simulink model "MIL4L3_SW6_V1_20220211"  (R2018b)
settings: Solver=FixedStepAuto  StartTime=0.0  StopTime=inf  FixedStep=0.001  RelTol=1e-3
PreLoadFcn:
  | A0_MILtest;
undefined symbols (not defined in the file or in its folder): Clb_ICADirect_LaneDisp_StateFive, Clb_ICADirect_LaneDisp_StateFour, Clb_ICADirect_LaneDisp_StateOne, Clb_ICADirect_LaneDisp_StateThree, Clb_ICADirect_LaneDisp_StateTwo, Clb_ICADirect_LaneDisp_StateZero, Clb_ICADirect_LaneDispSW, Clb_ICADirect_TrnLghtsCom_Switch, Clb_ICADirect_TrnLghtsCom_Value, Clb_ICADirect_TrnLghtsCrtl_Inhb, IMAP_Clb_ACU_Driver_Belt, IMAP_Clb_ACU_Driver_Belt_Over, IMAP_Clb_ACU_Passenger_Belt, IMAP_Clb_ACU_Passenger_Belt_Over, IMAP_Clb_ACU_RearLeft_Belt, IMAP_Clb_ACU_RearLeft_Belt_Over, IMAP_Clb_ACU_RearMiddle_Belt, IMAP_Clb_ACU_RearMiddle_Belt_Over, IMAP_Clb_ACU_RearRight_Belt, IMAP_Clb_ACU_RearRight_Belt_Over, IMAP_Clb_AEB_Switch, IMAP_Clb_AEB_Switch_Over, IMAP_Clb_ALC_TLC_Mode, IMAP_Clb_ALC_TLC_Mode_Over, IMAP_Clb_BCM_Battery_Voltage, IMAP_Clb_BCM_Battery_Voltage_Over, IMAP_Clb_BCM_BrakeLamp_State, IMAP_Clb_BCM_BrakeLamp_State_Over, IMAP_Clb_BCM_CHMSL_Status, IMAP_Clb_BCM_CHMSL_Status_Over, IMAP_Clb_BCM_Door_Lock_State, IMAP_Clb_BCM_Door_Lock_State_Over, IMAP_Clb_BCM_FrontWiper_State, IMAP_Clb_BCM_FrontWiper_State_Over, IMAP_Clb_BCM_FrontWiper_Switch, IMAP_Clb_BCM_FrontWiper_Switch_Over, IMAP_Clb_BCM_HazardLamp, IMAP_Clb_BCM_HazardLamp_Over, IMAP_Clb_BCM_HazardLamp_Switch, IMAP_Clb_BCM_HazardLamp_Switch_Over, IMAP_Clb_BCM_HighBeam_State, IMAP_Clb_BCM_HighBeam_State_Over, IMAP_Clb_BCM_Ignition_State, IMAP_Clb_BCM_Ignition_State_Over, IMAP_Clb_BCM_IHBC_Enabled, IMAP_Clb_BCM_IHBC_Enabled_Over, IMAP_Clb_BCM_Left_Light, IMAP_Clb_BCM_Left_Light_Over, IMAP_Clb_BCM_LeftTurn_Switch, IMAP_Clb_BCM_LeftTurn_Switch_Over, IMAP_Clb_BCM_LF_Door_State, IMAP_Clb_BCM_LF_Door_State_Over, IMAP_Clb_BCM_LowBeam_State, IMAP_Clb_BCM_LowBeam_State_Over, IMAP_Clb_BCM_LR_Door_State, IMAP_Clb_BCM_LR_Door_State_Over, IMAP_Clb_BCM_RF_Door_State, IMAP_Clb_BCM_RF_Door_State_Over, IMAP_Clb_BCM_Right_Light, IMAP_Clb_BCM_Right_Light_Over ... (+547)
libraries: CarMaker4SL x2153, simulink x292, dspstat3 x3, canmsglib x2, simulink_extras x1
(part 12 of 52)

== system MIL4L3_SW6_V1_20220211/CarMaker/VehicleControl/FunctionDataLog/AEB ==
  Bus Selector : BusSelector  OutputSignals=IMAPve_d_AEB_Switch,IMAPve_d_FCW_Switch,IMAPve_d_FCW_Sensitivity
  Bus Selector1 : BusSelector  OutputSignals=IMAPve_g_ESC_LatAcc,IMAPve_g_ESC_YawRate,IMAPve_d_ESC_YawRate_Valid,IMAPve_g_ESC_VehSpd,IMAPve_g_ESC_LonAcc,IMAPve_d_ESC_LonAcc_Valid,IMAPve_g_ESC_Brake_Press,IMAPve_g_ESC_Static_Slope,IMAPve_g_ESC_DySlope_Accuracy,IMAPve_g_ESC_DySlope
  Bus Selector10 : BusSelector  OutputSignals=IMAPve_d_ESC_ABS_Valid
  Bus Selector11 : BusSelector  OutputSignals=IMAPve_d_EMS_AccPedal_Fault
  Bus Selector2 : BusSelector  OutputSignals=IMAPve_g_SW_Angle,IMAPve_g_SW_Angle_Speed
  Bus Selector3 : BusSelector  OutputSignals=IMAPve_d_BCM_Left_Light,IMAPve_d_BCM_Right_Light,IMAPve_d_BCM_Opening_State
  Bus Selector4 : BusSelector  OutputSignals=IMAPve_g_EMS_RealPedal,IMAPve_d_ESC_Veh_Standstill,IMAPve_d_TCU_Actual_Gear
  Bus Selector5 : BusSelector  OutputSignals=IMAPve_d_BCM_Ignition_State,IMAPve_d_ACU_Driver_Belt,IMAPve_d_SWS_Fault_Code,IMAPve_d_SWS_Failure_Status,IMAPve_d_ESC_OFF,IMAPve_d_ESC_AlarmSig,IMAPve_d_ESC_ESC_Active,IMAPve_d_ESC_MSR_Active,IMAPve_d_ESC_TCS_Active,IMAPve_d_ESC_VehSpd_Valid,IMAPve_d_Brake_Pedal_Fault,IMAPve_d_ESC_ABS_Active,IMAPve_d_ESC_FL_WheelPulVal,IMAPve_d_ESC_FR_WheelPulVal,IMAPve_d_ESC_RL_WheelPulVal,IMAPve_d_ESC_RR_WheelPulVal,IMAPve_d_TCU_AT_Failure,IMAPve_d_EMS_Engine_Status,IMAPve_d_ESC_AEB_Status,IMAPve_d_ESC_AEB_Available,IMAPve_d_ESC_AEB_Active,IMAPve_d_BCM_FrontWiper_State,IMAPve_d_BCM_CHMSL_Status,IMAPve_d_BCM_BrakeLamp_State,IMAPve_d_ACU_Passenger_Belt,IMAPve_d_EMS_Brake_Pedal,IMAPve_d_EPB_Status,IMAPve_d_ESC_Drive_Direction,IMAPve_d_ESC_Hold_State,IMAPve_d_Radar_State,IMAPve_d_Signal_Time_Stamp,IMAPve_d_Time_System_Clock
  Bus Selector6 : BusSelector  OutputSignals=IMAPve_d_Sensor_Status,IMAPve_d_LF_Radar_Status,IMAPve_d_RF_Radar_Status,IMAPve_d_LR_Radar_Status,IMAPve_d_RR_Radar_Status,IMAPve_d_Fusion_Status,IMAPve_g_Fusion_Time_Stamp,IMAPve_d_obj_Num,IMAPva_d_obj_id,IMAPva_g_obj_pos_x,IMAPva_g_obj_pos_y,IMAPva_g_obj_vel_x,IMAPva_g_obj_vel_y,IMAPva_g_obj_acc_x,IMAPva_g_obj_acc_y,IMAPva_g_obj_pos_var_x,IMAPva_g_obj_pos_var_y,IMAPva_g_obj_pos_var_xy,IMAPva_g_obj_width,IMAPva_g_obj_length,IMAPva_d_obj_class,IMAPva_d_obj_lane,IMAPva_d_obj_status,IMAPva_d_obj_age,IMAPva_d_obj_TurnLight,IMAPva_d_obj_BrakeLight,IMAPva_d_obj_MotionStatus,IMAPve_d_Camera_Signal_Fault,IMAPve_d_Radar_Status,IMAPve_d_Camera_Status
  Bus Selector7 : BusSelector  OutputSignals=FDMMve_d_AebFcnConf,FDMMve_d_SignalTStamp
  Bus Selector8 : BusSelector  Commented=on  OutputSignals=JABSve_d_Switching,JABSve_a_DecelReq,JABSve_d_FltStatus,JABSve_d_AlertReq,JABSve_d_HapticAlarm,JABSve_d_Tips,JABSve_d_DbSignalTStamp
  Bus Selector9 : BusSelector  OutputSignals=IMAPve_d_ORI_CIPV_ID,IMAPve_d_ORI_Obj_Num,IMAPva_g_ORI_Probability,IMAPva_d_ORI_Obj_Class,IMAPva_d_ORI_Obj_Motion,IMAPva_g_ORI_Obj_RelVel,IMAPva_g_ORI_Obj_LongDis,IMAPva_d_ORI_Obj_Lane,IMAPva_g_ORI_Obj_LAngle,IMAPva_g_ORI_Obj_RAngle,IMAPva_g_ORI_Obj_Width,IMAPva_d_ORI_Obj_ID
  BusCreator : BusCreator  Inputs=109
  Data Type Conversion{,1..23,27..32} (30 alike) : DataTypeConversion
  From21 : From  Commented=on  GotoTag=JA_output
  Ground : Ground
  To Workspace : ToWorkspace  VariableName=AEBDataLog  SaveFormat=Timeseries  SampleTime=-1
  wires:
  [MDD_deceleration_type] -> BusCreator/107
  Bus Selector11/1 -> BusCreator/109  "<IMAPve_d_EMS_AccPedal_Fault>"
  [IMAP_bsPTState] -> Bus Selector11/1
  [IMAP_State] -> Bus Selector10/1
  Bus Selector9/12 -> BusCreator/105  "<IMAPva_d_ORI_Obj_ID>"
  Bus Selector9/11 -> BusCreator/104  "<IMAPva_g_ORI_Obj_Width>"
  Bus Selector9/10 -> BusCreator/103  "<IMAPva_g_ORI_Obj_RAngle>"
  Bus Selector9/9 -> BusCreator/102  "<IMAPva_g_ORI_Obj_LAngle>"
  Bus Selector9/8 -> BusCreator/101  "<IMAPva_d_ORI_Obj_Lane>"
  Bus Selector9/7 -> BusCreator/100  "<IMAPva_g_ORI_Obj_LongDis>"
  Bus Selector9/6 -> BusCreator/99  "<IMAPva_g_ORI_Obj_RelVel>"
  Bus Selector9/5 -> BusCreator/98  "<IMAPva_d_ORI_Obj_Motion>"
  Bus Selector9/4 -> BusCreator/97  "<IMAPva_d_ORI_Obj_Class>"
  Bus Selector9/3 -> BusCreator/96  "<IMAPva_g_ORI_Probability>"
  Bus Selector9/2 -> BusCreator/95  "<IMAPve_d_ORI_Obj_Num>"
  Bus Selector9/1 -> BusCreator/94  "<IMAPve_d_ORI_CIPV_ID>"
  [IMAP_ORI_obj] -> Bus Selector9/1
  [IMAPve_d_APA_AutoPark_WorkSt] -> BusCreator/108  "IMAPve_d_APA_AutoPark_WorkSt"
  Bus Selector10/1 -> BusCreator/106  "<IMAPve_d_ESC_ABS_Valid>"
  Bus Selector8/7 -> BusCreator/90  "<JABSve_d_DbSignalTStamp>"
  Ground/1 -> BusCreator/93
  Bus Selector7/2 -> BusCreator/92  "<FDMMve_d_SignalTStamp>"
  Bus Selector7/1 -> BusCreator/91  "<FDMMve_d_AebFcnConf>"
  Bus Selector8/6 -> BusCreator/89  "<JABSve_d_Tips>"
  Bus Selector8/5 -> BusCreator/88  "<JABSve_d_HapticAlarm>"
  Bus Selector8/4 -> BusCreator/87  "<JABSve_d_AlertReq>"
  Bus Selector8/3 -> BusCreator/86  "<JABSve_d_FltStatus>"
  Data Type Conversion32/1 -> BusCreator/83
  Bus Selector6/30 -> Data Type Conversion32/1  "<IMAPve_d_Camera_Status>"
  Data Type Conversion31/1 -> BusCreator/82
  Bus Selector6/29 -> Data Type Conversion31/1  "<IMAPve_d_Radar_Status>"
  Data Type Conversion30/1 -> BusCreator/81
  Bus Selector6/28 -> Data Type Conversion30/1  "<IMAPve_d_Camera_Signal_Fault>"
  Data Type Conversion29/1 -> BusCreator/80
  Bus Selector6/27 -> Data Type Conversion29/1  "<IMAPva_d_obj_MotionStatus>"
  Data Type Conversion28/1 -> BusCreator/79
  Bus Selector6/26 -> Data Type Conversion28/1  "<IMAPva_d_obj_BrakeLight>"
  Data Type Conversion27/1 -> BusCreator/78
  Bus Selector6/25 -> Data Type Conversion27/1  "<IMAPva_d_obj_TurnLight>"
  Data Type Conversion23/1 -> BusCreator/77
  Data Type Conversion22/1 -> BusCreator/76
  Data Type Conversion21/1 -> BusCreator/75
  Data Type Conversion20/1 -> BusCreator/74
  Data Type Conversion19/1 -> BusCreator/73
  Data Type Conversion18/1 -> BusCreator/72
  Data Type Conversion17/1 -> BusCreator/71
  Data Type Conversion16/1 -> BusCreator/70
  Data Type Conversion15/1 -> BusCreator/69
  Data Type Conversion14/1 -> BusCreator/68
  Data Type Conversion13/1 -> BusCreator/67
  Data Type Conversion12/1 -> BusCreator/66
  Data Type Conversion11/1 -> BusCreator/65
  Data Type Conversion10/1 -> BusCreator/64
  Data Type Conversion9/1 -> BusCreator/63
  Data Type Conversion8/1 -> BusCreator/62
  Data Type Conversion7/1 -> BusCreator/61
  Data Type Conversion6/1 -> BusCreator/60
  Data Type Conversion5/1 -> BusCreator/59
  Data Type Conversion4/1 -> BusCreator/58
  Data Type Conversion3/1 -> BusCreator/57
  Data Type Conversion2/1 -> BusCreator/56
  Data Type Conversion1/1 -> BusCreator/55
  Data Type Conversion/1 -> BusCreator/54
  Bus Selector5/32 -> BusCreator/53  "<IMAPve_d_Time_System_Clock>"
  Bus Selector5/31 -> BusCreator/52  "<IMAPve_d_Signal_Time_Stamp>"
  Bus Selector5/30 -> BusCreator/51  "<IMAPve_d_Radar_State>"
  Bus Selector5/29 -> BusCreator/50  "<IMAPve_d_ESC_Hold_State>"
  Bus Selector5/28 -> BusCreator/49  "<IMAPve_d_ESC_Drive_Direction>"
  Bus Selector5/27 -> BusCreator/48  "<IMAPve_d_EPB_Status>"
  Bus Selector5/26 -> BusCreator/47  "<IMAPve_d_EMS_Brake_Pedal>"
  Bus Selector5/25 -> BusCreator/46  "<IMAPve_d_ACU_Passenger_Belt>"
  Bus Selector5/24 -> BusCreator/45  "<IMAPve_d_BCM_BrakeLamp_State>"
  Bus Selector5/23 -> BusCreator/44  "<IMAPve_d_BCM_CHMSL_Status>"
  Bus Selector5/22 -> BusCreator/43  "<IMAPve_d_BCM_FrontWiper_State>"
  Bus Selector5/21 -> BusCreator/42  "<IMAPve_d_ESC_AEB_Active>"
  Bus Selector5/20 -> BusCreator/41  "<IMAPve_d_ESC_AEB_Available>"
  Bus Selector5/19 -> BusCreator/40  "<IMAPve_d_ESC_AEB_Status>"
  Bus Selector5/18 -> BusCreator/39  "<IMAPve_d_EMS_Engine_Status>"
  Bus Selector5/17 -> BusCreator/38  "<IMAPve_d_TCU_AT_Failure>"
  Bus Selector5/16 -> BusCreator/37  "<IMAPve_d_ESC_RR_WheelPulVal>"
  Bus Selector5/15 -> BusCreator/36  "<IMAPve_d_ESC_RL_WheelPulVal>"
  Bus Selector5/14 -> BusCreator/35  "<IMAPve_d_ESC_FR_WheelPulVal>"
  Bus Selector5/13 -> BusCreator/34  "<IMAPve_d_ESC_FL_WheelPulVal>"
  Bus Selector5/12 -> BusCreator/33  "<IMAPve_d_ESC_ABS_Active>"
  Bus Selector5/10 -> BusCreator/31  "<IMAPve_d_ESC_VehSpd_Valid>"
  Bus Selector5/11 -> BusCreator/32  "<IMAPve_d_Brake_Pedal_Fault>"
  Bus Selector5/9 -> BusCreator/30  "<IMAPve_d_ESC_TCS_Active>"
  Bus Selector5/8 -> BusCreator/29  "<IMAPve_d_ESC_MSR_Active>"
  Bus Selector5/7 -> BusCreator/28  "<IMAPve_d_ESC_ESC_Active>"
  Bus Selector5/6 -> BusCreator/27  "<IMAPve_d_ESC_AlarmSig>"
  Bus Selector5/5 -> BusCreator/26  "<IMAPve_d_ESC_OFF>"
  Bus Selector5/4 -> BusCreator/25  "<IMAPve_d_SWS_Failure_Status>"
  Bus Selector5/3 -> BusCreator/24  "<IMAPve_d_SWS_Fault_Code>"
  Bus Selector5/2 -> BusCreator/23  "<IMAPve_d_ACU_Driver_Belt>"
  Bus Selector5/1 -> BusCreator/22  "<IMAPve_d_BCM_Ignition_State>"
  Bus Selector4/3 -> BusCreator/21  "<IMAPve_d_TCU_Actual_Gear>"
  Bus Selector4/2 -> BusCreator/20  "<IMAPve_d_ESC_Veh_Standstill>"
  Bus Selector4/1 -> BusCreator/19  "<IMAPve_g_EMS_RealPedal>"
  Bus Selector3/3 -> BusCreator/18  "<IMAPve_d_BCM_Opening_State>"
  Bus Selector3/2 -> BusCreator/17  "<IMAPve_d_BCM_Right_Light>"
  Bus Selector3/1 -> BusCreator/16  "<IMAPve_d_BCM_Left_Light>"
  Bus Selector2/2 -> BusCreator/15  "<IMAPve_g_SW_Angle_Speed>"
  Bus Selector2/1 -> BusCreator/14  "<IMAPve_g_SW_Angle>"
  Bus Selector1/10 -> BusCreator/13  "<IMAPve_g_ESC_DySlope>"
  Bus Selector1/9 -> BusCreator/12  "<IMAPve_g_ESC_DySlope_Accuracy>"
  Bus Selector1/8 -> BusCreator/11  "<IMAPve_g_ESC_Static_Slope>"
  Bus Selector1/7 -> BusCreator/10  "<IMAPve_g_ESC_Brake_Press>"
  Bus Selector1/6 -> BusCreator/9  "<IMAPve_d_ESC_LonAcc_Valid>"
  Bus Selector1/5 -> BusCreator/8  "<IMAPve_g_ESC_LonAcc>"
  Bus Selector1/4 -> BusCreator/7  "<IMAPve_g_ESC_VehSpd>"
  Bus Selector6/13 -> Data Type Conversion12/1  "<IMAPva_g_obj_vel_y>"
  Bus Selector6/12 -> Data Type Conversion11/1  "<IMAPva_g_obj_vel_x>"
  Bus Selector6/11 -> Data Type Conversion10/1  "<IMAPva_g_obj_pos_y>"
  Bus Selector6/10 -> Data Type Conversion9/1  "<IMAPva_g_obj_pos_x>"
  Bus Selector6/9 -> Data Type Conversion8/1  "<IMAPva_d_obj_id>"
  Bus Selector6/8 -> Data Type Conversion7/1  "<IMAPve_d_obj_Num>"
  Bus Selector6/7 -> Data Type Conversion6/1  "<IMAPve_g_Fusion_Time_Stamp>"
  Bus Selector6/6 -> Data Type Conversion5/1  "<IMAPve_d_Fusion_Status>"
  Bus Selector6/5 -> Data Type Conversion4/1  "<IMAPve_d_RR_Radar_Status>"
  Bus Selector6/4 -> Data Type Conversion3/1  "<IMAPve_d_LR_Radar_Status>"
  Bus Selector6/14 -> Data Type Conversion13/1  "<IMAPva_g_obj_acc_x>"
  Bus Selector6/15 -> Data Type Conversion14/1  "<IMAPva_g_obj_acc_y>"
  Bus Selector6/16 -> Data Type Conversion15/1  "<IMAPva_g_obj_pos_var_x>"
  Bus Selector6/17 -> Data Type Conversion16/1  "<IMAPva_g_obj_pos_var_y>"
  Bus Selector6/18 -> Data Type Conversion17/1  "<IMAPva_g_obj_pos_var_xy>"
  Bus Selector6/19 -> Data Type Conversion18/1  "<IMAPva_g_obj_width>"
  Bus Selector6/20 -> Data Type Conversion19/1  "<IMAPva_g_obj_length>"
  Bus Selector6/21 -> Data Type Conversion20/1  "<IMAPva_d_obj_class>"
  Bus Selector6/22 -> Data Type Conversion21/1  "<IMAPva_d_obj_lane>"
  Bus Selector6/23 -> Data Type Conversion22/1  "<IMAPva_d_obj_status>"
  Bus Selector6/24 -> Data Type Conversion23/1  "<IMAPva_d_obj_age>"
  Bus Selector6/3 -> Data Type Conversion2/1  "<IMAPve_d_RF_Radar_Status>"
  Bus Selector6/2 -> Data Type Conversion1/1  "<IMAPve_d_LF_Radar_Status>"
  Bus Selector6/1 -> Data Type Conversion/1  "<IMAPve_d_Sensor_Status>"
  Bus Selector1/3 -> BusCreator/6  "<IMAPve_d_ESC_YawRate_Valid>"
  Bus Selector1/2 -> BusCreator/5  "<IMAPve_g_ESC_YawRate>"
  Bus Selector1/1 -> BusCreator/4  "<IMAPve_g_ESC_LatAcc>"
  From21/1 -> Bus Selector8/1
  [FDMM_output] -> Bus Selector7/1
  [IMAP_Fusion_Sig] -> Bus Selector6/1
  [IMAP_State] -> Bus Selector5/1
  [IMAP_bsPTState] -> Bus Selector4/1
  [IMAP_BESRx] -> Bus Selector3/1
  [IMAP_SWARx] -> Bus Selector2/1
  [IMAP_VehMovRx] -> Bus Selector1/1
  [IMAP_MP5Rx] -> Bus Selector/1
  Bus Selector/3 -> BusCreator/3  "<IMAPve_d_FCW_Sensitivity>"
  Bus Selector/2 -> BusCreator/2  "<IMAPve_d_FCW_Switch>"
  Bus Selector8/2 -> BusCreator/85  "<JABSve_a_DecelReq>"
  Bus Selector8/1 -> BusCreator/84  "<JABSve_d_Switching>"
  Bus Selector/1 -> BusCreator/1  "<IMAPve_d_AEB_Switch>"
  BusCreator/1 -> To Workspace/1

== system MIL4L3_SW6_V1_20220211/CarMaker/VehicleControl/FunctionDataLog/ELK ==
  Bus Selector : BusSelector  OutputSignals=IMAPve_d_LKA_Mode,IMAPve_d_ELK_Switch
  Bus Selector1 : BusSelector  OutputSignals=IMAPve_g_EMS_RealPedal,IMAPve_d_TCU_Actual_Gear,IMAPve_d_TCU_Target_Gear
  Bus Selector10 : BusSelector  OutputSignals=IMAPve_g_SW_Angle,IMAPve_g_SW_Angle_Speed
  Bus Selector11 : BusSelector  OutputSignals=IMAPve_g_ESC_LatAcc,IMAPve_g_ESC_YawRate,IMAPve_g_ESC_UnYawRate,IMAPve_g_ESC_VehSpd,IMAPve_g_ESC_LonAcc,IMAPve_g_ESC_Brake_Press
  Bus Selector12 : BusSelector  OutputSignals=IMAPve_d_BCM_Ignition_State,IMAPve_d_ACU_Driver_Belt,IMAPve_d_SWS_Fault_Code,IMAPve_d_SWS_Failure_Status,IMAPve_d_ESC_OFF,IMAPve_d_ESC_AlarmSig,IMAPve_d_ESC_ESC_Active,IMAPve_d_ESC_MSR_Active,IMAPve_d_ESC_TCS_Active,IMAPve_d_ESC_ABS_Active,IMAPve_d_ESC_FL_WheelPulVal,IMAPve_d_ESC_FR_WheelPulVal,IMAPve_d_ESC_RL_WheelPulVal,IMAPve_d_ESC_RR_WheelPulVal,IMAPve_d_ESC_AEB_Active,IMAPve_d_BCM_FrontWiper_State,IMAPve_d_BCM_HighBeam_State,IMAPve_d_ESC_Drive_Direction,IMAPve_d_EPS_Steer_Hold_State,IMAPve_d_Time_System_Clock
  Bus Selector13 : BusSelector  OutputSignals=IMAPva_g_ORI_Obj_AbsAx,IMAPva_g_ORI_Obj_AbsAy,IMAPva_g_ORI_Obj_RelVely,IMAPva_g_ORI_Obj_LateralDis,IMAPva_g_ORI_Obj_ExistProb,IMAPva_g_ORI_Obj_ClassProb,IMAPve_d_ORI_L0_ID,IMAPve_g_ORI_L0_ExistProb,IMAPve_g_ORI_L0_TypeConf,IMAPve_d_ORI_R0_ID,IMAPve_g_ORI_R0_ExistProb,IMAPve_g_ORI_R0_TypeConf,IMAPve_d_ORI_L1_ID,IMAPve_g_ORI_L1_ExistProb,IMAPve_g_ORI_L1_TypeConf,IMAPve_d_ORI_R1_ID,IMAPve_g_ORI_R1_ExistProb,IMAPve_g_ORI_R1_TypeConf,IMAPve_d_ORI_RoadedgeL0_ID,IMAPve_g_ORI_RoadedgeL0_ExistProb,IMAPve_g_ORI_RoadedgeL0_C1,IMAPve_g_ORI_RoadedgeL0_C0,IMAPve_g_ORI_RoadedgeL0_C3,IMAPve_g_ORI_RoadedgeL0_C2,IMAPve_d_ORI_RoadedgeL0_Type,IMAPve_g_ORI_RoadedgeR0_C1,IMAPve_g_ORI_RoadedgeR0_C0,IMAPve_g_ORI_RoadedgeR0_C3,IMAPve_g_ORI_RoadedgeR0_C2,IMAPve_d_ORI_RoadedgeR0_Type
  Bus Selector2 : BusSelector  OutputSignals=IMAPve_d_ORI_CIPV_ID,IMAPve_d_ORI_Obj_Num,IMAPva_g_ORI_Probability,IMAPva_d_ORI_Obj_Class,IMAPva_d_ORI_Obj_Motion,IMAPva_g_ORI_Obj_RelVel,IMAPva_g_ORI_Obj_LongDis,IMAPva_d_ORI_Obj_Lane,IMAPva_g_ORI_Obj_LAngle,IMAPva_g_ORI_Obj_RAngle,IMAPva_g_ORI_Obj_Width,IMAPva_d_ORI_Obj_ID
  Bus Selector3 : BusSelector  OutputSignals=IMAPve_d_ORI_Lane_Valid,IMAPve_d_ORI_Lane_ConsArea,IMAPve_d_ORI_Lane_RoadType,IMAPve_g_ORI_L0_C3,IMAPve_g_ORI_L0_C2,IMAPve_g_ORI_L0_C1,IMAPve_g_ORI_L0_C0,IMAPve_d_ORI_L0_Q,IMAPve_d_ORI_L0_Type,IMAPve_g_ORI_L0_VR,IMAPve_g_ORI_L0_TLC,IMAPve_g_ORI_L0_W,IMAPve_d_ORI_L0_LC,IMAPve_g_ORI_L1_C3,IMAPve_g_ORI_L1_C2,IMAPve_g_ORI_L1_C1,IMAPve_g_ORI_L1_C0,IMAPve_d_ORI_L1_Q,IMAPve_d_ORI_L1_Type,IMAPve_g_ORI_L1_VR,IMAPve_g_ORI_L1_TLC,IMAPve_g_ORI_L1_W,IMAPve_d_ORI_L1_LC,IMAPve_g_ORI_R0_C3,IMAPve_g_ORI_R0_C2,IMAPve_g_ORI_R0_C1,IMAPve_g_ORI_R0_C0,IMAPve_d_ORI_R0_Q,IMAPve_d_ORI_R0_LT,IMAPve_g_ORI_R0_VR,IMAPve_g_ORI_R0_TLC,IMAPve_g_ORI_R0_W,IMAPve_d_ORI_R0_LC,IMAPve_g_ORI_R1_C3,IMAPve_g_ORI_R1_C2,IMAPve_g_ORI_R1_C1,IMAPve_g_ORI_R1_C0,IMAPve_d_ORI_R1_Q,IMAPve_d_ORI_R1_LT,IMAPve_g_ORI_R1_VR,IMAPve_g_ORI_R1_TLC,IMAPve_g_ORI_R1_W,IMAPve_d_ORI_R1_LC
  Bus Selector4 : BusSelector  OutputSignals=IMAPve_d_Sensor_Status,IMAPve_d_LF_Radar_Status,IMAPve_d_RF_Radar_Status,IMAPve_d_LR_Radar_Status,IMAPve_d_RR_Radar_Status,IMAPve_d_Fusion_Status,IMAPve_g_Fusion_Time_Stamp,IMAPve_d_obj_Num,IMAPva_d_obj_id,IMAPva_g_obj_pos_x,IMAPva_g_obj_pos_y,IMAPva_g_obj_vel_x,IMAPva_g_obj_vel_y,IMAPva_g_obj_acc_x,IMAPva_g_obj_acc_y,IMAPva_g_obj_pos_var_x,IMAPva_g_obj_pos_var_y,IMAPva_g_obj_pos_var_xy,IMAPva_g_obj_width,IMAPva_g_obj_length,IMAPva_d_obj_class,IMAPva_d_obj_lane,IMAPva_d_obj_status,IMAPva_d_obj_TurnLight,IMAPva_d_obj_BrakeLight,IMAPva_d_obj_MotionStatus,IMAPve_d_Lane_Valid,IMAPve_d_Road_Type,IMAPve_d_ConsArea,IMAPve_g_L0_C0,IMAPve_g_L0_C1,IMAPve_g_L0_C2,IMAPve_g_L0_C3,IMAPve_g_L0_VR,IMAPve_d_L0_Q,IMAPve_d_L0_Type,IMAPve_g_L0_Confidence,IMAPve_g_L0_W,IMAPve_g_L0_TLC,IMAPve_d_L0_LC,IMAPve_g_R0_C0,IMAPve_g_R0_C1,IMAPve_g_R0_C2,IMAPve_g_R0_C3,IMAPve_g_R0_VR,IMAPve_d_R0_Q,IMAPve_d_R0_Type,IMAPve_g_R0_Confidence,IMAPve_g_R0_W,IMAPve_g_R0_TLC,IMAPve_d_R0_LC,IMAPve_g_L1_C0,IMAPve_g_L1_C1,IMAPve_g_L1_C2,IMAPve_g_L1_C3,IMAPve_g_L1_VR,IMAPve_d_L1_Q,IMAPve_d_L1_Type,IMAPve_g_L1_Confidence,IMAPve_g_L1_W,IMAPve_g_L1_TLC,IMAPve_d_L1_LC,IMAPve_g_R1_C0,IMAPve_g_R1_C1,IMAPve_g_R1_C2,IMAPve_g_R1_C3,IMAPve_g_R1_VR,IMAPve_d_R1_Q,IMAPve_d_R1_Type,IMAPve_g_R1_Confidence,IMAPve_g_R1_W,IMAPve_g_R1_TLC,IMAPve_d_R1_LC,IMAPve_g_L0_C0_Back,IMAPve_g_L0_C1_Back,IMAPve_g_L0_C2_Back,IMAPve_g_L0_C3_Back,IMAPve_g_L0_Range_Back,IMAPve_g_L0_C0_FR_Pred,IMAPve_g_L0_C1_FR_Pred,IMAPve_g_L0_C2_FR_Pred,IMAPve_g_L0_Range_FR_Pred,IMAPve_g_R0_C0_Back,IMAPve_g_R0_C1_Back,IMAPve_g_R0_C2_Back,IMAPve_g_R0_C3_Back,IMAPve_g_R0_Range_Back,IMAPve_g_R0_C0_FR_Pred,IMAPve_g_R0_C1_FR_Pred,IMAPve_g_R0_C2_FR_Pred,IMAPve_g_R0_Range_FR_Pred,IMAPve_g_L1_C0_Back,IMAPve_g_L1_C1_Back,IMAPve_g_L1_C2_Back,IMAPve_g_L1_C3_Back,IMAPve_g_L1_Range_Back,IMAPve_g_L1_C0_FR_Pred,IMAPve_g_L1_C1_FR_Pred,IMAPve_g_L1_C2_FR_Pred,IMAPve_g_L1_Range_FR_Pred,IMAPve_g_R1_C0_Back,IMAPve_g_R1_C1_Back,IMAPve_g_R1_C2_Back,IMAPve_g_R1_C3_Back,IMAPve_g_R1_Range_Back,IMAPve_g_R1_C0_FR_Pred,IMAPve_g_R1_C1_FR_Pred,IMAPve_g_R1_C2_FR_Pred,IMAPve_g_R1_Range_FR_Pred,IMAPve_d_Sign_ISA_Value,IMAPve_d_TSR_Sign_Type,IMAPve_d_Camera_Signal_Fault,IMAPve_d_Radar_Status,IMAPve_d_Camera_Status
  Bus Selector5 : BusSelector  OutputSignals=IMAPve_d_EPS_SteeringAngle_Flag,IMAPve_g_EPS_SteeringAngle,IMAPve_d_EPS_Driver_Override,IMAPve_d_EPS_Driver_Active_ESA
  Bus Selector6 : BusSelector  OutputSignals=FDMMve_d_ElkFcnConf,FDMMve_d_SignalTStamp
  Bus Selector7 : BusSelector  OutputSignals=IMAPve_d_Signal_Time_Stamp
  Bus Selector8 : BusSelector  OutputSignals=IMAPve_d_EPS_LKA_State,IMAPve_g_EPS_SW_Trq,IMAPve_d_EPS_Error_State
  Bus Selector9 : BusSelector  OutputSignals=IMAPve_d_BCM_HazardLamp,IMAPve_d_BCM_Left_Light,IMAPve_d_BCM_Right_Light,IMAPve_d_BCM_Opening_State
  BusCreator : BusCreator  Inputs=249
  Constant : Constant  Commented=on  Value=0
  Constant1 : Constant  Commented=on  Value=0
  Constant2 : Constant  Commented=on  Value=0
  Data Type Conversion : DataTypeConversion  Commented=on
  Data Type Conversion1 : DataTypeConversion  Commented=on
  Data Type Conversion2 : DataTypeConversion  Commented=on
  Ground : Ground
  Ground1 : Ground
  To Workspace : ToWorkspace  VariableName=ELKDataLog  SaveFormat=Timeseries  SampleTime=-1
  wires:
  Ground1/1 -> BusCreator/249  "Runable_functionstep"
  Bus Selector13/30 -> BusCreator/248  "<IMAPve_d_ORI_RoadedgeR0_Type>"
  Bus Selector13/29 -> BusCreator/247  "<IMAPve_g_ORI_RoadedgeR0_C2>"
  Bus Selector13/28 -> BusCreator/246  "<IMAPve_g_ORI_RoadedgeR0_C3>"
  Bus Selector13/27 -> BusCreator/245  "<IMAPve_g_ORI_RoadedgeR0_C0>"
  Bus Selector13/26 -> BusCreator/244  "<IMAPve_g_ORI_RoadedgeR0_C1>"
  Bus Selector13/25 -> BusCreator/243  "<IMAPve_d_ORI_RoadedgeL0_Type>"
  Bus Selector13/24 -> BusCreator/242  "<IMAPve_g_ORI_RoadedgeL0_C2>"
  Bus Selector13/23 -> BusCreator/241  "<IMAPve_g_ORI_RoadedgeL0_C3>"
  Bus Selector13/22 -> BusCreator/240  "<IMAPve_g_ORI_RoadedgeL0_C0>"
  Bus Selector13/21 -> BusCreator/239  "<IMAPve_g_ORI_RoadedgeL0_C1>"
  Bus Selector13/20 -> BusCreator/238  "<IMAPve_g_ORI_RoadedgeL0_ExistProb>"
  Bus Selector13/19 -> BusCreator/237  "<IMAPve_d_ORI_RoadedgeL0_ID>"
  Bus Selector13/18 -> BusCreator/236  "<IMAPve_g_ORI_R1_TypeConf>"
  Bus Selector13/17 -> BusCreator/235  "<IMAPve_g_ORI_R1_ExistProb>"
  Bus Selector13/16 -> BusCreator/234  "<IMAPve_d_ORI_R1_ID>"
  Bus Selector13/15 -> BusCreator/233  "<IMAPve_g_ORI_L1_TypeConf>"
  Bus Selector13/14 -> BusCreator/232  "<IMAPve_g_ORI_L1_ExistProb>"
  Bus Selector13/13 -> BusCreator/231  "<IMAPve_d_ORI_L1_ID>"
  Bus Selector13/12 -> BusCreator/230  "<IMAPve_g_ORI_R0_TypeConf>"
  Bus Selector13/11 -> BusCreator/229  "<IMAPve_g_ORI_R0_ExistProb>"
  Bus Selector13/10 -> BusCreator/228  "<IMAPve_d_ORI_R0_ID>"
  Bus Selector13/9 -> BusCreator/227  "<IMAPve_g_ORI_L0_TypeConf>"
  Bus Selector13/8 -> BusCreator/226  "<IMAPve_g_ORI_L0_ExistProb>"
  Bus Selector13/7 -> BusCreator/225  "<IMAPve_d_ORI_L0_ID>"
  Bus Selector13/6 -> BusCreator/224  "<IMAPva_g_ORI_Obj_ClassProb>"
  Bus Selector13/5 -> BusCreator/223  "<IMAPva_g_ORI_Obj_ExistProb>"
  Bus Selector13/4 -> BusCreator/222  "<IMAPva_g_ORI_Obj_LateralDis>"
  Bus Selector13/3 -> BusCreator/221  "<IMAPva_g_ORI_Obj_RelVely>"
  Bus Selector13/2 -> BusCreator/220  "<IMAPva_g_ORI_Obj_AbsAy>"
  Bus Selector13/1 -> BusCreator/219  "<IMAPva_g_ORI_Obj_AbsAx>"
  [ORI_AddSW4] -> Bus Selector13/1
  Ground/1 -> BusCreator/218
  [busNew] -> Bus Selector5/1
  Bus Selector4/114 -> BusCreator/217  "<IMAPve_d_Camera_Status>"
  Bus Selector4/113 -> BusCreator/216  "<IMAPve_d_Radar_Status>"
  Bus Selector4/112 -> BusCreator/215  "<IMAPve_d_Camera_Signal_Fault>"
  Bus Selector4/111 -> BusCreator/214  "<IMAPve_d_TSR_Sign_Type>"
  Bus Selector4/110 -> BusCreator/213  "<IMAPve_d_Sign_ISA_Value>"
  Bus Selector4/109 -> BusCreator/212  "<IMAPve_g_R1_Range_FR_Pred>"
  Bus Selector4/108 -> BusCreator/211  "<IMAPve_g_R1_C2_FR_Pred>"
  Bus Selector4/107 -> BusCreator/210  "<IMAPve_g_R1_C1_FR_Pred>"
  Bus Selector4/106 -> BusCreator/209  "<IMAPve_g_R1_C0_FR_Pred>"
  Bus Selector4/105 -> BusCreator/208  "<IMAPve_g_R1_Range_Back>"
  Bus Selector4/104 -> BusCreator/207  "<IMAPve_g_R1_C3_Back>"
  Bus Selector4/103 -> BusCreator/206  "<IMAPve_g_R1_C2_Back>"
  Bus Selector4/102 -> BusCreator/205  "<IMAPve_g_R1_C1_Back>"
  Bus Selector4/101 -> BusCreator/204  "<IMAPve_g_R1_C0_Back>"
  Bus Selector4/100 -> BusCreator/203  "<IMAPve_g_L1_Range_FR_Pred>"
  Bus Selector4/99 -> BusCreator/202  "<IMAPve_g_L1_C2_FR_Pred>"
  Bus Selector4/98 -> BusCreator/201  "<IMAPve_g_L1_C1_FR_Pred>"
  Bus Selector4/97 -> BusCreator/200  "<IMAPve_g_L1_C0_FR_Pred>"
  Bus Selector4/96 -> BusCreator/199  "<IMAPve_g_L1_Range_Back>"
  Bus Selector4/95 -> BusCreator/198  "<IMAPve_g_L1_C3_Back>"
  Bus Selector4/94 -> BusCreator/197  "<IMAPve_g_L1_C2_Back>"
  Bus Selector4/93 -> BusCreator/196  "<IMAPve_g_L1_C1_Back>"
  Bus Selector4/92 -> BusCreator/195  "<IMAPve_g_L1_C0_Back>"
  Bus Selector4/91 -> BusCreator/194  "<IMAPve_g_R0_Range_FR_Pred>"
  Bus Selector4/90 -> BusCreator/193  "<IMAPve_g_R0_C2_FR_Pred>"
  Bus Selector4/89 -> BusCreator/192  "<IMAPve_g_R0_C1_FR_Pred>"
  Bus Selector4/88 -> BusCreator/191  "<IMAPve_g_R0_C0_FR_Pred>"
  Bus Selector4/87 -> BusCreator/190  "<IMAPve_g_R0_Range_Back>"
  Bus Selector4/86 -> BusCreator/189  "<IMAPve_g_R0_C3_Back>"
  Bus Selector4/85 -> BusCreator/188  "<IMAPve_g_R0_C2_Back>"
  Bus Selector4/84 -> BusCreator/187  "<IMAPve_g_R0_C1_Back>"
  Bus Selector4/83 -> BusCreator/186  "<IMAPve_g_R0_C0_Back>"
  Bus Selector4/82 -> BusCreator/185  "<IMAPve_g_L0_Range_FR_Pred>"
  Bus Selector4/81 -> BusCreator/184  "<IMAPve_g_L0_C2_FR_Pred>"
  Bus Selector4/80 -> BusCreator/183  "<IMAPve_g_L0_C1_FR_Pred>"
  Bus Selector4/79 -> BusCreator/182  "<IMAPve_g_L0_C0_FR_Pred>"
  Bus Selector4/78 -> BusCreator/181  "<IMAPve_g_L0_Range_Back>"
  Bus Selector4/77 -> BusCreator/180  "<IMAPve_g_L0_C3_Back>"
  Bus Selector4/76 -> BusCreator/179  "<IMAPve_g_L0_C2_Back>"
  Bus Selector4/75 -> BusCreator/178  "<IMAPve_g_L0_C1_Back>"
  Bus Selector4/74 -> BusCreator/177  "<IMAPve_g_L0_C0_Back>"
  Bus Selector4/73 -> BusCreator/176  "<IMAPve_d_R1_LC>"
  Bus Selector4/72 -> BusCreator/175  "<IMAPve_g_R1_TLC>"
  Bus Selector4/71 -> BusCreator/174  "<IMAPve_g_R1_W>"
  Bus Selector4/70 -> BusCreator/173  "<IMAPve_g_R1_Confidence>"
  Bus Selector4/69 -> BusCreator/172  "<IMAPve_d_R1_Type>"
  Bus Selector4/68 -> BusCreator/171  "<IMAPve_d_R1_Q>"
  Bus Selector4/67 -> BusCreator/170  "<IMAPve_g_R1_VR>"
  Bus Selector4/66 -> BusCreator/169  "<IMAPve_g_R1_C3>"
  Bus Selector4/65 -> BusCreator/168  "<IMAPve_g_R1_C2>"
  Bus Selector4/64 -> BusCreator/167  "<IMAPve_g_R1_C1>"
  Bus Selector4/63 -> BusCreator/166  "<IMAPve_g_R1_C0>"
  Bus Selector4/62 -> BusCreator/165  "<IMAPve_d_L1_LC>"
  Bus Selector4/61 -> BusCreator/164  "<IMAPve_g_L1_TLC>"
  Bus Selector4/60 -> BusCreator/163  "<IMAPve_g_L1_W>"
  Bus Selector4/59 -> BusCreator/162  "<IMAPve_g_L1_Confidence>"
  Bus Selector4/58 -> BusCreator/161  "<IMAPve_d_L1_Type>"
  Bus Selector4/57 -> BusCreator/160  "<IMAPve_d_L1_Q>"
  Bus Selector4/56 -> BusCreator/159  "<IMAPve_g_L1_VR>"
  Bus Selector4/55 -> BusCreator/158  "<IMAPve_g_L1_C3>"
  Bus Selector4/54 -> BusCreator/157  "<IMAPve_g_L1_C2>"
  Bus Selector4/53 -> BusCreator/156  "<IMAPve_g_L1_C1>"
  Bus Selector4/52 -> BusCreator/155  "<IMAPve_g_L1_C0>"
  Bus Selector4/51 -> BusCreator/154  "<IMAPve_d_R0_LC>"
  Bus Selector4/50 -> BusCreator/153  "<IMAPve_g_R0_TLC>"
  Bus Selector4/49 -> BusCreator/152  "<IMAPve_g_R0_W>"
  Bus Selector4/48 -> BusCreator/151  "<IMAPve_g_R0_Confidence>"
  Bus Selector4/47 -> BusCreator/150  "<IMAPve_d_R0_Type>"
  Bus Selector4/46 -> BusCreator/149  "<IMAPve_d_R0_Q>"
  Bus Selector4/45 -> BusCreator/148  "<IMAPve_g_R0_VR>"
  Bus Selector4/44 -> BusCreator/147  "<IMAPve_g_R0_C3>"
  Bus Selector4/43 -> BusCreator/146  "<IMAPve_g_R0_C2>"
  Bus Selector4/42 -> BusCreator/145  "<IMAPve_g_R0_C1>"
  Bus Selector4/41 -> BusCreator/144  "<IMAPve_g_R0_C0>"
  Bus Selector4/40 -> BusCreator/143  "<IMAPve_d_L0_LC>"
  Bus Selector4/39 -> BusCreator/142  "<IMAPve_g_L0_TLC>"
  Bus Selector4/38 -> BusCreator/141  "<IMAPve_g_L0_W>"
  Bus Selector4/37 -> BusCreator/140  "<IMAPve_g_L0_Confidence>"
  Bus Selector4/36 -> BusCreator/139  "<IMAPve_d_L0_Type>"
  Bus Selector4/35 -> BusCreator/138  "<IMAPve_d_L0_Q>"
  Bus Selector4/34 -> BusCreator/137  "<IMAPve_g_L0_VR>"
  Bus Selector4/33 -> BusCreator/136  "<IMAPve_g_L0_C3>"
  Bus Selector4/32 -> BusCreator/135  "<IMAPve_g_L0_C2>"
  Bus Selector4/31 -> BusCreator/134  "<IMAPve_g_L0_C1>"
  Bus Selector4/30 -> BusCreator/133  "<IMAPve_g_L0_C0>"
  Bus Selector4/29 -> BusCreator/132  "<IMAPve_d_ConsArea>"
  Bus Selector4/28 -> BusCreator/131  "<IMAPve_d_Road_Type>"
  Bus Selector4/27 -> BusCreator/130  "<IMAPve_d_Lane_Valid>"
  Bus Selector4/26 -> BusCreator/129  "<IMAPva_d_obj_MotionStatus>"
  Bus Selector4/25 -> BusCreator/128  "<IMAPva_d_obj_BrakeLight>"
  Bus Selector4/24 -> BusCreator/127  "<IMAPva_d_obj_TurnLight>"
  Bus Selector4/23 -> BusCreator/126  "<IMAPva_d_obj_status>"
  Bus Selector4/22 -> BusCreator/125  "<IMAPva_d_obj_lane>"
  Bus Selector4/21 -> BusCreator/124  "<IMAPva_d_obj_class>"
  Bus Selector4/20 -> BusCreator/123  "<IMAPva_g_obj_length>"
  Bus Selector4/19 -> BusCreator/122  "<IMAPva_g_obj_width>"
  Bus Selector4/18 -> BusCreator/121  "<IMAPva_g_obj_pos_var_xy>"
  Bus Selector4/17 -> BusCreator/120  "<IMAPva_g_obj_pos_var_y>"
  Bus Selector4/16 -> BusCreator/119  "<IMAPva_g_obj_pos_var_x>"
  Bus Selector4/15 -> BusCreator/118  "<IMAPva_g_obj_acc_y>"
  Bus Selector4/14 -> BusCreator/117  "<IMAPva_g_obj_acc_x>"
  Bus Selector4/13 -> BusCreator/116  "<IMAPva_g_obj_vel_y>"
  Bus Selector4/12 -> BusCreator/115  "<IMAPva_g_obj_vel_x>"
  Bus Selector4/11 -> BusCreator/114  "<IMAPva_g_obj_pos_y>"
  Bus Selector4/10 -> BusCreator/113  "<IMAPva_g_obj_pos_x>"
  Bus Selector4/9 -> BusCreator/112  "<IMAPva_d_obj_id>"
  Bus Selector4/8 -> BusCreator/111  "<IMAPve_d_obj_Num>"
  Bus Selector4/7 -> BusCreator/110  "<IMAPve_g_Fusion_Time_Stamp>"
  Bus Selector4/6 -> BusCreator/109  "<IMAPve_d_Fusion_Status>"
  Bus Selector4/5 -> BusCreator/108  "<IMAPve_d_RR_Radar_Status>"
  Bus Selector4/4 -> BusCreator/107  "<IMAPve_d_LR_Radar_Status>"
  Bus Selector4/3 -> BusCreator/106  "<IMAPve_d_RF_Radar_Status>"
  Bus Selector4/2 -> BusCreator/105  "<IMAPve_d_LF_Radar_Status>"
  Bus Selector4/1 -> BusCreator/104  "<IMAPve_d_Sensor_Status>"
  Bus Selector3/43 -> BusCreator/103  "<IMAPve_d_ORI_R1_LC>"
  Bus Selector3/42 -> BusCreator/102  "<IMAPve_g_ORI_R1_W>"
  Bus Selector3/41 -> BusCreator/101  "<IMAPve_g_ORI_R1_TLC>"
  Bus Selector3/40 -> BusCreator/100  "<IMAPve_g_ORI_R1_VR>"
  Bus Selector3/39 -> BusCreator/99  "<IMAPve_d_ORI_R1_LT>"
  Bus Selector3/38 -> BusCreator/98  "<IMAPve_d_ORI_R1_Q>"
  Bus Selector3/37 -> BusCreator/97  "<IMAPve_g_ORI_R1_C0>"
  Bus Selector3/36 -> BusCreator/96  "<IMAPve_g_ORI_R1_C1>"
  Bus Selector3/35 -> BusCreator/95  "<IMAPve_g_ORI_R1_C2>"
  Bus Selector3/34 -> BusCreator/94  "<IMAPve_g_ORI_R1_C3>"
  Bus Selector3/33 -> BusCreator/93  "<IMAPve_d_ORI_R0_LC>"
  Bus Selector3/32 -> BusCreator/92  "<IMAPve_g_ORI_R0_W>"
  Bus Selector3/31 -> BusCreator/91  "<IMAPve_g_ORI_R0_TLC>"
  Bus Selector3/30 -> BusCreator/90  "<IMAPve_g_ORI_R0_VR>"
  Bus Selector3/29 -> BusCreator/89  "<IMAPve_d_ORI_R0_LT>"
  Bus Selector3/28 -> BusCreator/88  "<IMAPve_d_ORI_R0_Q>"
  Bus Selector3/27 -> BusCreator/87  "<IMAPve_g_ORI_R0_C0>"
  Bus Selector3/26 -> BusCreator/86  "<IMAPve_g_ORI_R0_C1>"
  Bus Selector3/25 -> BusCreator/85  "<IMAPve_g_ORI_R0_C2>"
  Bus Selector3/24 -> BusCreator/84  "<IMAPve_g_ORI_R0_C3>"
  Bus Selector3/23 -> BusCreator/83  "<IMAPve_d_ORI_L1_LC>"
  Bus Selector3/22 -> BusCreator/82  "<IMAPve_g_ORI_L1_W>"
  Bus Selector3/21 -> BusCreator/81  "<IMAPve_g_ORI_L1_TLC>"
  Bus Selector3/20 -> BusCreator/80  "<IMAPve_g_ORI_L1_VR>"
  Bus Selector3/19 -> BusCreator/79  "<IMAPve_d_ORI_L1_Type>"
  Bus Selector5/4 -> BusCreator/21  "<IMAPve_d_EPS_Driver_Active_ESA>"
  Bus Selector5/3 -> BusCreator/20  "<IMAPve_d_EPS_Driver_Override>"
  Bus Selector5/2 -> BusCreator/19  "<IMAPve_g_EPS_SteeringAngle>"
  Bus Selector5/1 -> BusCreator/18  "<IMAPve_d_EPS_SteeringAngle_Flag>"
  [IMAPve_d_APA_AutoPark_WorkSt] -> BusCreator/4  "IMAPve_d_APA_AutoPark_WorkSt"
  Constant2/1 -> Data Type Conversion2/1
  Constant1/1 -> Data Type Conversion1/1
  Constant/1 -> Data Type Conversion/1
  [IMAP_Fusion_Sig] -> Bus Selector4/1
  Bus Selector3/18 -> BusCreator/78  "<IMAPve_d_ORI_L1_Q>"
  Bus Selector3/17 -> BusCreator/77  "<IMAPve_g_ORI_L1_C0>"
  Bus Selector3/16 -> BusCreator/76  "<IMAPve_g_ORI_L1_C1>"
  Bus Selector3/15 -> BusCreator/75  "<IMAPve_g_ORI_L1_C2>"
  Bus Selector3/14 -> BusCreator/74  "<IMAPve_g_ORI_L1_C3>"
  Bus Selector3/13 -> BusCreator/73  "<IMAPve_d_ORI_L0_LC>"
  Bus Selector3/12 -> BusCreator/72  "<IMAPve_g_ORI_L0_W>"
  Bus Selector3/11 -> BusCreator/71  "<IMAPve_g_ORI_L0_TLC>"
  Bus Selector3/10 -> BusCreator/70  "<IMAPve_g_ORI_L0_VR>"
  Bus Selector3/9 -> BusCreator/69  "<IMAPve_d_ORI_L0_Type>"
  Bus Selector3/8 -> BusCreator/68  "<IMAPve_d_ORI_L0_Q>"
  Bus Selector3/7 -> BusCreator/67  "<IMAPve_g_ORI_L0_C0>"
  Bus Selector3/6 -> BusCreator/66  "<IMAPve_g_ORI_L0_C1>"
  Bus Selector3/5 -> BusCreator/65  "<IMAPve_g_ORI_L0_C2>"
  Bus Selector3/4 -> BusCreator/64  "<IMAPve_g_ORI_L0_C3>"
  Bus Selector3/3 -> BusCreator/63  "<IMAPve_d_ORI_Lane_RoadType>"
  Bus Selector3/2 -> BusCreator/62  "<IMAPve_d_ORI_Lane_ConsArea>"
  Bus Selector3/1 -> BusCreator/61  "<IMAPve_d_ORI_Lane_Valid>"
  [IMAP_ORI_Lane] -> Bus Selector3/1
  Bus Selector2/12 -> BusCreator/60  "<IMAPva_d_ORI_Obj_ID>"
  Bus Selector2/11 -> BusCreator/59  "<IMAPva_g_ORI_Obj_Width>"
  Bus Selector2/10 -> BusCreator/58  "<IMAPva_g_ORI_Obj_RAngle>"
  Bus Selector2/9 -> BusCreator/57  "<IMAPva_g_ORI_Obj_LAngle>"
  Bus Selector2/8 -> BusCreator/56  "<IMAPva_d_ORI_Obj_Lane>"
  Bus Selector2/7 -> BusCreator/55  "<IMAPva_g_ORI_Obj_LongDis>"
  Bus Selector2/6 -> BusCreator/54  "<IMAPva_g_ORI_Obj_RelVel>"
  Bus Selector2/5 -> BusCreator/53  "<IMAPva_d_ORI_Obj_Motion>"
  Bus Selector2/4 -> BusCreator/52  "<IMAPva_d_ORI_Obj_Class>"
  Bus Selector2/3 -> BusCreator/51  "<IMAPva_g_ORI_Probability>"
  Bus Selector2/2 -> BusCreator/50  "<IMAPve_d_ORI_Obj_Num>"
  Bus Selector2/1 -> BusCreator/49  "<IMAPve_d_ORI_CIPV_ID>"
  [IMAP_ORI_obj] -> Bus Selector2/1
  Bus Selector12/20 -> BusCreator/48  "<IMAPve_d_Time_System_Clock>"
  Bus Selector12/19 -> BusCreator/47  "<IMAPve_d_EPS_Steer_Hold_State>"
  Bus Selector12/18 -> BusCreator/46  "<IMAPve_d_ESC_Drive_Direction>"
  Bus Selector12/17 -> BusCreator/45  "<IMAPve_d_BCM_HighBeam_State>"
  Bus Selector12/16 -> BusCreator/44  "<IMAPve_d_BCM_FrontWiper_State>"
  Bus Selector12/15 -> BusCreator/43  "<IMAPve_d_ESC_AEB_Active>"
  Bus Selector12/14 -> BusCreator/42  "<IMAPve_d_ESC_RR_WheelPulVal>"
  Bus Selector12/13 -> BusCreator/41  "<IMAPve_d_ESC_RL_WheelPulVal>"
  Bus Selector12/12 -> BusCreator/40  "<IMAPve_d_ESC_FR_WheelPulVal>"
  Bus Selector12/11 -> BusCreator/39  "<IMAPve_d_ESC_FL_WheelPulVal>"
  Bus Selector12/10 -> BusCreator/38  "<IMAPve_d_ESC_ABS_Active>"
  Bus Selector12/9 -> BusCreator/37  "<IMAPve_d_ESC_TCS_Active>"
  Bus Selector12/8 -> BusCreator/36  "<IMAPve_d_ESC_MSR_Active>"
  Bus Selector12/7 -> BusCreator/35  "<IMAPve_d_ESC_ESC_Active>"
  Bus Selector12/6 -> BusCreator/34  "<IMAPve_d_ESC_AlarmSig>"
  Bus Selector12/5 -> BusCreator/33  "<IMAPve_d_ESC_OFF>"
  Bus Selector12/3 -> BusCreator/31  "<IMAPve_d_SWS_Fault_Code>"
  Bus Selector12/4 -> BusCreator/32  "<IMAPve_d_SWS_Failure_Status>"
  Bus Selector12/2 -> BusCreator/30  "<IMAPve_d_ACU_Driver_Belt>"
  Bus Selector12/1 -> BusCreator/29  "<IMAPve_d_BCM_Ignition_State>"
  [IMAP_State] -> Bus Selector12/1, Bus Selector7/1
  Bus Selector1/3 -> BusCreator/28  "<IMAPve_d_TCU_Target_Gear>"
  Bus Selector1/2 -> BusCreator/27  "<IMAPve_d_TCU_Actual_Gear>"
  Bus Selector1/1 -> BusCreator/26  "<IMAPve_g_EMS_RealPedal>"
  [IMAP_bsPTState] -> Bus Selector1/1
  Bus Selector11/6 -> BusCreator/15  "<IMAPve_g_ESC_Brake_Press>"
  Bus Selector11/5 -> BusCreator/14  "<IMAPve_g_ESC_LonAcc>"
  Bus Selector11/4 -> BusCreator/13  "<IMAPve_g_ESC_VehSpd>"
  Bus Selector11/3 -> BusCreator/12  "<IMAPve_g_ESC_UnYawRate>"
  Bus Selector11/2 -> BusCreator/11  "<IMAPve_g_ESC_YawRate>"
  Bus Selector11/1 -> BusCreator/10  "<IMAPve_g_ESC_LatAcc>"
  [IMAP_VehMovRx] -> Bus Selector11/1
  Bus Selector10/2 -> BusCreator/17  "<IMAPve_g_SW_Angle_Speed>"
  Bus Selector10/1 -> BusCreator/16  "<IMAPve_g_SW_Angle>"
  [IMAP_SWARx] -> Bus Selector10/1
  Bus Selector9/4 -> BusCreator/25  "<IMAPve_d_BCM_Opening_State>"
  Bus Selector9/3 -> BusCreator/24  "<IMAPve_d_BCM_Right_Light>"
  Bus Selector9/2 -> BusCreator/23  "<IMAPve_d_BCM_Left_Light>"
  Bus Selector9/1 -> BusCreator/22  "<IMAPve_d_BCM_HazardLamp>"
  [IMAP_BESRx] -> Bus Selector9/1
  Bus Selector8/3 -> BusCreator/9  "<IMAPve_d_EPS_Error_State>"
  Bus Selector8/2 -> BusCreator/8  "<IMAPve_g_EPS_SW_Trq>"
  Bus Selector8/1 -> BusCreator/7  "<IMAPve_d_EPS_LKA_State>"
  [IMAP_EPSRx] -> Bus Selector8/1
  Bus Selector7/1 -> BusCreator/3  "<IMAPve_d_Signal_Time_Stamp>"
  Bus Selector/2 -> BusCreator/6  "<IMAPve_d_ELK_Switch>"
  Bus Selector6/2 -> BusCreator/2  "<FDMMve_d_SignalTStamp>"
  Bus Selector6/1 -> BusCreator/1  "<FDMMve_d_ElkFcnConf>"
  [FDMM_output] -> Bus Selector6/1
  Bus Selector/1 -> BusCreator/5  "<IMAPve_d_LKA_Mode>"
  [IMAP_MP5Rx] -> Bus Selector/1
  BusCreator/1 -> To Workspace/1
